simulink model "oven_0_US"  (R2015b)
settings: Solver=ode45  StartTime=0.0  StopTime=5000  RelTol=1e-3
values from neighbouring files (symbols this model uses):
  a = 0.5    [oven_parameters_US.m]
  G = 0.8    [oven_parameters_US.m]
  K = 15    [oven_parameters_US.m]
  Ki = 0.01    [oven_parameters_US.m]
  Kp = 10    [oven_parameters_US.m]
  T = 2500    [oven_parameters_US.m]
libraries: simulink x1
settings Model: Creator=Ivan  LastModifiedBy=Ivan
settings DataIOCC: SaveFormat=Array  SignalLoggingSaveFormat=ModelDataLogs
settings OptimizationCC: ExpressionDepthLimit=2147483647  InitFltsAndDblsToZero=on
settings DebuggingCC: SaveWithParameterizedLinksMsg=none  UnderspecifiedInitializationDetection=Classic  MergeDetectMultiDrivingBlocksExec=none  SignalResolutionControl=TryResolveAllWithWarning  SolverPrmCheckMsg=warning  MultiTaskDSMMsg=warning  MultiTaskCondExecSysMsg=none  FcnCallInpInsideContextMsg=UseLocalSettings  StateNameClashWarn=warning
settings HardwareCC: ProdBitPerPointer=32  ProdLargestAtomicFloat=None  ProdIntDivRoundTo=Undefined  ProdEndianess=Unspecified  ProdWordSize=32  ProdHWDeviceType=32-bit Generic
settings GRTTargetCC: TargetFcnLib=ansi_tfl_tmw.mat  GeneratePreprocessorConditionals=Disable all  CombineOutputUpdateFcns=off  GRTInterface=on
settings ConfigComp: CovModelRefEnable=Off

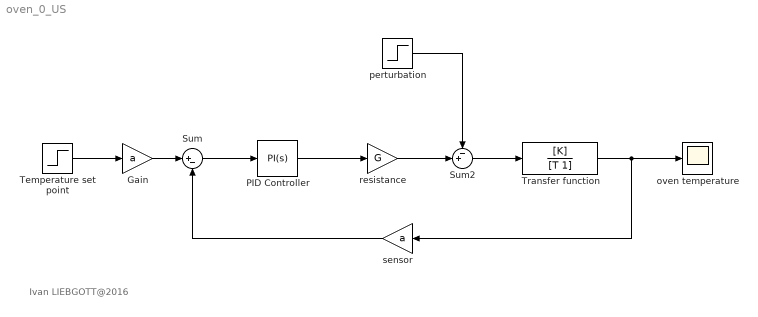
== system oven_0_US ==
  note: Ivan LIEBGOTT@2016
  Gain : Gain  Gain=a
  PID Controller : simulink/Continuous/PID Controller  Controller=PI  TimeDomain=Continuous-time  SampleTime=-1  IntegratorMethod=Forward Euler  FilterMethod=Forward Euler  Form=Parallel  UseFilter=on  ControllerParametersSource=internal  P=Kp  I=Ki  D=0  N=100  InitialConditionSource=internal  InitialConditionForIntegrator=0  InitialConditionForFilter=0  ExternalReset=none  LimitOutput=off  UpperSaturationLimit=inf  LowerSaturationLimit=-inf  LinearizeAsGain=on  AntiWindupMode=none  Kb=1  TrackingMode=off  Kt=1  PParamMin=[]  PParamMax=[]  IParamMin=[]  IParamMax=[]  DParamMin=[]  DParamMax=[]  NParamMin=[]  NParamMax=[]  KbParamMin=[]  KbParamMax=[]  KtParamMin=[]  KtParamMax=[]  POutMin=[]  POutMax=[]  IOutMin=[]  IOutMax=[]  DOutMin=[]  DOutMax=[]  NOutMin=[]  NOutMax=[]  KbOutMin=[]  KbOutMax=[]  KtOutMin=[]  KtOutMax=[]  IntegratorOutMin=[]  IntegratorOutMax=[]  FilterOutMin=[]  FilterOutMax=[]  SumOutMin=[]  SumOutMax=[]  SumI1OutMin=[]  SumI1OutMax=[]  SumI2OutMin=[]  SumI2OutMax=[]  SumI3OutMin=[]  SumI3OutMax=[]  SumDOutMin=[]  SumDOutMax=[]  SaturationOutMin=[]  SaturationOutMax=[]  IntegratorContinuousStateAttributes=''  IntegratorStateMustResolveToSignalObject=off  IntegratorRTWStateStorageClass=Auto  FilterContinuousStateAttributes=''  FilterStateMustResolveToSignalObject=off  FilterRTWStateStorageClass=Auto  DifferentiatorICPrevScaledInput=0  DifferentiatorOutMin=[]  DifferentiatorOutMax=[]
  Sum : Sum  Inputs=|+-
  Sum2 : Sum  Inputs=-+|
  Temperature set point : Step  Time=0  After=100  SampleTime=0
  "Transfer function " : TransferFcn  Numerator=[K]  Denominator=[T 1]
  oven temperature : Scope
  perturbation : Step  Time=600  After=50  SampleTime=0
  resistance : Gain  Gain=G
  sensor : Gain  Gain=a
  wires:
  sensor/1 -> Sum/2
  Sum/1 -> PID Controller/1
  Temperature set point/1 -> Gain/1
  Gain/1 -> Sum/1
  "Transfer function "/1 -> sensor/1, oven temperature/1
  resistance/1 -> Sum2/2
  Sum2/1 -> "Transfer function "/1
  perturbation/1 -> Sum2/1
  PID Controller/1 -> resistance/1
